simulink model "VCU_SW_1"  (R2023b)
settings: Solver=FixedStepDiscrete  StartTime=0.0  StopTime=inf  FixedStep=1e-2  RelTol=1e-3
PreLoadFcn:
  | RTWConfigurationCB('preloadfcn', bdroot);
InitFcn:
  | loadvar_ttc500
undefined symbols (not defined in the file): BrkPedalTypes, CabMovModeTypes, cFuseTempSensAcc_X, cFuseTempSensAcc_Y, cFuseTempSensVal_X, cFuseTempSensVal_Y, cTMSTempSensVal_X, cTMSTempSensVal_Y, cTransferCaseSpeedRatio, diag_state, DoorsPositionTypes, dP_filter_Y, DriverOccClassSystemTypes, ErrorValueTypes, fatal_error_callback, IO_ADC_NO_RANGE, LadderStatusTypes, pAnalogCabRotSensAcc, pAnalogCabRotSensMaxVolt, pAnalogCabRotSensMinVolt, pAnalogCabRotSensRange, pAnalogCabRotSensZeroVolt, pBrkActivePress, pCabTiltSensAcc, pCabTiltSensMaxCur, pCabTiltSensMinCur, pDistanceCorrection, pECANManual_BPNEnable, pECANManual_BPNEnabler_Flag, pFilterSensAccRes, pHDirMaxDiffFrq, pHDirSensHighLvl, pHDirSensLowLvl, pMainGearRatio, pMaxFilterSensRes, pMaxFirstPedalSensValue, pMaxFuseTempSensRes, pMaxPressLoss, pMaxPressSensCurrent, pMaxPressValue, pMaxPressValueHydMotAndPump, pMaxPressValueParkDrain, pMaxSecondPedalSensValue, pMaxTempSensVoltage, pMaxTempValue, pMaxTMSTempSensRes, pMinFilterSensRes, pMinFirstPedalSensValue, pMinFuseTempSensRes, pMinPressLoss, pMinPressSensCurrent, pMinPressValue, pMinSecondPedalSensValue, pMinTempSensVoltage, pMinTempValue, pMinTMSTempSensRes, pMotorRingTeethNum, pPedalSensAccuracyPct, pPedalSensAccuracyVolt, pPressLossTreshhold ... (+20)
libraries: TTlibrary x270, canmsglib x127, simulink x88
(part 12 of 19)

== system VCU_SW_1/InputLayer/InputInterfaces/AnalogInput/AIProc10msec/WasherTiltPumpTrans ==
  Abs : Abs  SaturateOnIntegerOverflow=off
  Constant12 : Constant  Value=pWasherTiltPumpTransSensMaxVolt
  Constant13 : Constant  Value=pWasherTiltPumpTransSensMinVolt
  Constant14 : Constant  Value=pWasherTiltPumpTransSensAcc
  Data Store Read3 : DataStoreRead  DataStoreName=InputInterfaceData  DataStoreElements=InputInterfaceData.AI.washerTiltPumpTransSens  IndexOptions=Index vector (dialog)  Indices=1  OutputSizes=1
  Data Store Write14 : DataStoreWrite  DataStoreName=InputFunctionsData  DataStoreElements=InputFunctionsData.washerTiltPumpTransPct  IndexOptions=Index vector (dialog)  Indices=1  OutputSizes=1
  Data Store Write40 : DataStoreWrite  DataStoreName=UDSStruct  DataStoreElements=UDSStruct.washerTiltPumpTransSens  IndexOptions=Index vector (dialog)  Indices=1  OutputSizes=1
  Data Type Conversion : DataTypeConversion  OutDataTypeStr=uint16  SaturateOnIntegerOverflow=off  RndMeth=Floor
  getWasherTiltPumpTransSensDataFcn : MATLAB Function  TreatAsAtomicUnit=on
  wires:
  Data Type Conversion/1 -> Data Store Write40/1
  Abs/1 -> Data Type Conversion/1
  getWasherTiltPumpTransSensDataFcn/1(washerTiltPercent) -> Abs/1, Data Store Write14/1
  Constant13/1 -> getWasherTiltPumpTransSensDataFcn/3(minVolt)
  Constant14/1 -> getWasherTiltPumpTransSensDataFcn/4(accuracy)
  Constant12/1 -> getWasherTiltPumpTransSensDataFcn/2(maxVolt)
  Data Store Read3/1 -> getWasherTiltPumpTransSensDataFcn/1(washerTiltPumpTransSens)

== system VCU_SW_1/InputLayer/InputInterfaces/DigitalInput/Function-Call Subsystem/cabRotIndSensProc ==
  function : TriggerPort  TriggerType=function-call  VariantControl=Variant
  Constant1 : Constant  Value=pResetIndCabSensErr
  cabRotIndSensProc fcn : MATLAB Function  TreatAsAtomicUnit=on
  getIndRotSensData : Subsystem  TreatAsAtomicUnit=on
  setIndRotSensData : Subsystem  TreatAsAtomicUnit=on
  setIndSensErr : Subsystem  TreatAsAtomicUnit=on
  wires:
  Constant1/1 -> cabRotIndSensProc fcn/1(pResetIndCabSensErr)

== system VCU_SW_1/InputLayer/InputInterfaces/DigitalInput/Function-Call Subsystem2/cabRotIndSensProc ==
  function : TriggerPort  TriggerType=function-call  VariantControl=Variant
  Constant1 : Constant  Value=pResetIndCabSensErr
  cabRotIndSensProc fcn : MATLAB Function  TreatAsAtomicUnit=on
  getIndRotSensData : Subsystem  TreatAsAtomicUnit=on
  setIndRotSensData : Subsystem  TreatAsAtomicUnit=on
  setIndSensErr : Subsystem  TreatAsAtomicUnit=on
  wires:
  Constant1/1 -> cabRotIndSensProc fcn/1(pResetIndCabSensErr)

== system VCU_SW_1/InputLayer/InputInterfaces/PWDInput/PWDProc100msec/calcSpdSens ==
  calcSpdSensValue : TriggerPort  TriggerType=function-call  IsSimulinkFunction=on  FunctionName=calcSpdSensValue  FunctionVisibility=scoped  VariantControl=(inherit)
  MATLAB Function : MATLAB Function  TreatAsAtomicUnit=on
  teethNum : ArgIn  OutDataTypeStr=uint16  ArgumentName=teethNum
  sensFreq : ArgIn  Port=2  OutDataTypeStr=uint16  ArgumentName=sensFreq
  SpdValue : ArgOut  DisableCoverage=on  OutDataTypeStr=uint16  ArgumentName=SpdValue
  wires:
  sensFreq/1 -> MATLAB Function/1(sensFreq)
  teethNum/1 -> MATLAB Function/2(teethNum)
  MATLAB Function/1(Spd) -> SpdValue/1

== system VCU_SW_1/InputLayer/InputInterfaces/PWDInput/PWDProc100msec/validatePedalSensValue ==
  validateSpdSensValue : TriggerPort  TriggerType=function-call  IsSimulinkFunction=on  FunctionName=validateSpdSensValue  FunctionVisibility=scoped  VariantControl=(inherit)
  Ground : Ground
  MATLAB Function : MATLAB Function  TreatAsAtomicUnit=on
  fstValue : ArgIn  DisableCoverage=on  OutDataTypeStr=uint16  ArgumentName=fstValue
  secValue : ArgIn  Port=2  OutDataTypeStr=uint16  ArgumentName=secValue
  SpdVal : ArgOut  OutDataTypeStr=uint16  ArgumentName=SpdVal
  errorSts : ArgOut  Port=2  OutDataTypeStr=uint8  ArgumentName=errorSts
  wires:
  fstValue/1 -> MATLAB Function/1(firstSensValue)
  secValue/1 -> MATLAB Function/2(secondSensValue)
  Ground/1 -> errorSts/1
  MATLAB Function/1(SpdValue) -> SpdVal/1

== system VCU_SW_1/InputLayer/InputInterfaces/PWMCurrentInput/PWMCur10msecProc/Simulink Function ==
  ValveCurFBproc : TriggerPort  TriggerType=function-call  IsSimulinkFunction=on  FunctionName=ValveCurFBproc  FunctionVisibility=scoped  VariantControl=(inherit)
  MATLAB Function : MATLAB Function  TreatAsAtomicUnit=on
  pValveActiveCur : ArgIn  DisableCoverage=on  OutDataTypeStr=uint16  ArgumentName=pValveActiveCur
  curFB : ArgIn  Port=2  OutDataTypeStr=uint16  ArgumentName=curFB
  stt : ArgOut  DisableCoverage=on  OutDataTypeStr=Enum: StateModeTypes  ArgumentName=stt
  wires:
  MATLAB Function/1(stt) -> stt/1
  curFB/1 -> MATLAB Function/2(curFB)
  pValveActiveCur/1 -> MATLAB Function/1(pValveActiveCur)

== system VCU_SW_1/InputLayer/InputNetwork/InputCCAN/CCAN100msecProc1/CabMov buttons processing ==
  note: Main Fcns
  MATLAB Function : MATLAB Function  TreatAsAtomicUnit=on
  callRotFcn : Subsystem  TreatAsAtomicUnit=on
  callTiltFcn : Subsystem  TreatAsAtomicUnit=on

== system VCU_SW_1/InputLayer/InputNetwork/InputCCAN/CCAN100msecProc1/InputTransSelect ==
  Constant : Constant  Commented=on  Value=3  OutDataTypeStr=uint8
  Constant1 : Constant  Commented=on  Value=0  OutDataTypeStr=uint8
  Constant2 : Constant  Commented=on  Value=0  OutDataTypeStr=uint8
  Constant3 : Constant  Commented=on  OutDataTypeStr=uint8
  Data Store Read : DataStoreRead  DataStoreName=InputNetworkData  DataStoreElements=InputNetworkData.CCAN.TC1.Trans_Requested_Gear  IndexOptions=Index vector (dialog)  Indices=1  OutputSizes=1
  Data Store Read1 : DataStoreRead  DataStoreName=InputInterfaceData  DataStoreElements=InputInterfaceData.DI.selector_signal_1#InputInterfaceData.DI.selector_signal_2#InputInterfaceData.DI.selector_signal_3  IndexOptions=Index vector (dialog)  Indices=1  OutputSizes=1
  Data Store Write1 : DataStoreWrite  DataStoreName=InputFunctionsData  DataStoreElements=InputFunctionsData.LeverPosition  IndexOptions=Index vector (dialog)  Indices=1  OutputSizes=1
  Data Type Conversion : DataTypeConversion  Commented=on  OutDataTypeStr=Enum: StateModeTypes  SaturateOnIntegerOverflow=off  RndMeth=Floor
  Data Type Conversion1 : DataTypeConversion  Commented=on  OutDataTypeStr=Enum: StateModeTypes  SaturateOnIntegerOverflow=off  RndMeth=Floor
  Data Type Conversion2 : DataTypeConversion  Commented=on  OutDataTypeStr=Enum: StateModeTypes  SaturateOnIntegerOverflow=off  RndMeth=Floor
  Data Type Conversion3 : DataTypeConversion  Commented=on  OutDataTypeStr=Enum: LeverPosTypes  SaturateOnIntegerOverflow=off  RndMeth=Floor
  Function Caller1 : FunctionCaller  FunctionPrototype=LeverPos = calcLeverPos(TransReqGear,SelSig1,SelSig2,SelSig3)  InputArgumentSpecifications=<Enter example>  OutputArgumentSpecifications=<Enter example>
  calcLeverPos : Subsystem  TreatAsAtomicUnit=on
  wires:
  Data Store Read1/3 -> Function Caller1/4
  Data Store Read1/2 -> Function Caller1/3
  Data Store Read1/1 -> Function Caller1/2
  Data Store Read/1 -> Function Caller1/1
  Constant3/1 -> Data Type Conversion2/1
  Constant2/1 -> Data Type Conversion1/1
  Constant1/1 -> Data Type Conversion/1
  Constant/1 -> Data Type Conversion3/1
  Function Caller1/1 -> Data Store Write1/1

== system VCU_SW_1/InputLayer/InputNetwork/InputCCAN/CCAN100msecProc1/JoystickRot ==
  Data Store Read1 : DataStoreRead  DataStoreName=InputNetworkData  DataStoreElements=InputNetworkData.CCAN.BJM2.J2_Y_NeutralPosSts#InputNetworkData.CCAN.BJM2.J2_Y_BackNegPosSts#InputNetworkData.CCAN.BJM2.J2_Y_ForwPosSts#InputNetworkData.CCAN.BJM2.J2_Y_Pos  IndexOptions=Index vector (dialog)  Indices=1  OutputSizes=1
  Data Store Write1 : DataStoreWrite  DataStoreName=InputFunctionsData  DataStoreElements=InputFunctionsData.rotJoyPos  IndexOptions=Index vector (dialog)  Indices=1  OutputSizes=1
  Data Store Write2 : DataStoreWrite  DataStoreName=InputFunctionsData  DataStoreElements=InputFunctionsData.rotJoyDir  IndexOptions=Index vector (dialog)  Indices=1  OutputSizes=1
  MATLAB Function : MATLAB Function  TreatAsAtomicUnit=on
  wires:
  MATLAB Function/1(pos) -> Data Store Write1/1
  MATLAB Function/2(dir) -> Data Store Write2/1
  Data Store Read1/1 -> MATLAB Function/1(neutralPos)
  Data Store Read1/2 -> MATLAB Function/2(fwdPos)
  Data Store Read1/4 -> MATLAB Function/4(absPos)
  Data Store Read1/3 -> MATLAB Function/3(bckwsPos)

== system VCU_SW_1/InputLayer/InputNetwork/InputCCAN/GetCCAN1000msec/DD ==
  CAN_Unpack_PLC_StateM : canmsglib/CAN Unpack  MsgList=(none)  MsgName=DD  MsgIDType=Extended (29-bit identifier)  MsgIdentifier=419364094  MsgLength=8  SignalInfo={ 'FuelLevelTank1', '8', '8', 'LE', 'unsigned', 'Standard', '0', '0.4', '0', '0', '100'; 'FuelLevelTank2', '48', '8', 'LE', 'unsigned', 'Standard', '0', '0.4', '0', '0', '100'; 'WasherFluidLevel', '0', '8', 'LE', 'unsigned', 'Standard', '0', '0.4', '0', '0', '100' }  IDPort=off  TimestampPort=off  ErrorPort=off  RemotePort=off  LengthPort=off  StatusPort=off  ApplyMinMax=off
  DataStoreWrite_PLC_StateM : DataStoreWrite  DataStoreName=InputNetworkData  DataStoreElements=InputNetworkData.CCAN.DD.FuelLevelTank1#InputNetworkData.CCAN.DD.FuelLevelTank2#InputNetworkData.CCAN.DD.WasherFluidLevel  IndexOptions=Index vector (dialog)  Indices=1  OutputSizes=1
  Terminator : Terminator
  read_message_PLC_StateM : TTlibrary/CAN/read_message_name  channel=IO_CAN_CHANNEL_1  id_format=IO_CAN_EXT_FRAME  get_msg_info=off  message_names=there is no CAN Unpack blocks  message_info=|  id=419364094  ac_mask=536870911  retranslation=off  io_error=on  sample_time=-1
      | Message Name: DD
      |  Message ID Type: Extended (29-bit identifier)
      |  Message ID: 419364094
      settings: SourceProductName=TT control 500 series
  wires:
  read_message_PLC_StateM/2 -> Terminator/1  "handler_err_419364094"
  read_message_PLC_StateM/1 -> CAN_Unpack_PLC_StateM/1  "msg_419364094"
  CAN_Unpack_PLC_StateM/1 -> DataStoreWrite_PLC_StateM/1
  CAN_Unpack_PLC_StateM/2 -> DataStoreWrite_PLC_StateM/2
  CAN_Unpack_PLC_StateM/3 -> DataStoreWrite_PLC_StateM/3

== system VCU_SW_1/InputLayer/InputNetwork/InputCCAN/GetCCAN1000msec/Fuel Heater Data  ==
  CAN_Unpack_PLC_StateM : canmsglib/CAN Unpack  MsgList=(none)  MsgName=FuelHeaterData  MsgIDType=Extended (29-bit identifier)  MsgIdentifier=419377406  MsgLength=8  SignalInfo={ 'FuelHeaterValue', '0', '8', 'LE', 'unsigned', 'Standard', '0', '0.4', '0', '0', '100' }  IDPort=off  TimestampPort=off  ErrorPort=off  RemotePort=off  LengthPort=off  StatusPort=off  ApplyMinMax=off
  DataStoreWrite_PLC_StateM : DataStoreWrite  DataStoreName=InputNetworkData  DataStoreElements=InputNetworkData.CCAN.FuelHeaterData.FuelHeaterValue  IndexOptions=Index vector (dialog)  Indices=1  OutputSizes=1
  Terminator : Terminator
  read_message_PLC_StateM : TTlibrary/CAN/read_message_name  channel=IO_CAN_CHANNEL_1  id_format=IO_CAN_EXT_FRAME  get_msg_info=off  message_names=there is no CAN Unpack blocks  message_info=|  id=419377406  ac_mask=536870911  retranslation=off  io_error=on  sample_time=-1
      | Message Name: FuelHeaterData
      |  Message ID Type: Extended (29-bit identifier)
      |  Message ID: 419377406
      settings: SourceProductName=TT control 500 series
  wires:
  read_message_PLC_StateM/2 -> Terminator/1  "handler_err_419377406"
  read_message_PLC_StateM/1 -> CAN_Unpack_PLC_StateM/1  "msg_419377406"
  CAN_Unpack_PLC_StateM/1 -> DataStoreWrite_PLC_StateM/1

== system VCU_SW_1/InputLayer/InputNetwork/InputCCAN/GetCCAN1000msec/LCMD ==
  CAN_Unpack_PLC_StateM : canmsglib/CAN Unpack  MsgList=(none)  MsgName=LCMD  MsgIDType=Extended (29-bit identifier)  MsgIdentifier=217989381  MsgLength=8  SignalInfo={ 'CenterStopLightCmd', '18', '2', 'LE', 'unsigned', 'Standard', '0', '1', '0', '0', '3'; 'HighBeamHeadLightCmd', '6', '2', 'LE', 'unsigned', 'Standard', '0', '1', '0', '0', '3'; 'ImplOEMOpt1LightCmd', '50', '2', 'LE', 'unsigned', 'Standard', '0', '1', '0', '0', '3'; 'ImplOEMOpt2LightCmd', '48', '2', 'LE', 'unsigned', 'Standard', '0', '1', '0', '0', '3'; 'ImplRightFacingWrkLightCmd', '52', '2', 'LE', 'unsigned', 'Standard', '0', '1', '0', '0', '3'; 'ImplementMarkerLightCmd', '28', '2', 'LE', 'unsigned', 'Standard', '0', '1', '0', '0', '3'; 'LeftStopLightCmd', '22', '2', 'LE', 'unsigned', 'Standard', '0', '1', '0', '0', '3'; 'LeftTurnSignalLightsCmd', '14', '2', 'LE', 'unsigned', 'Standard', '0', '1', '0', '0', '3'; 'LowBeamHeadLightCmd', '4', '2', 'LE', 'unsigned', 'Standard', '0', '1', '0', '0', '3'; 'RightStopLightCmd', '20', '2', 'LE', 'unsigned', 'Standard', '0', '1', '0', '0', '3'; 'RightTurnSignalLightsCmd', '12', '2', 'LE', 'unsigned', 'Standard', '0', '1', '0', '0', '3'; 'RotatingBeaconLightCmd', '10', '2', 'LE', 'unsigned', 'Standard', '0', '1', '0', '0', '3'; 'RunLightCmd', '0', '2', 'LE', 'unsigned', 'Standard', '0', '1', '0', '0', '3'; 'TractorFrontFogLightsCmd', '8', '2', 'LE', 'unsigned', 'Standard', '0', '1', '0', '0', '3'; 'TrctrFrntHighMntdWrkLightsCmd', '46', '2', 'LE', 'unsigned', 'Standard', '0', '1', '0', '0', '3'; 'TrctrRearHighMntdWrkLightsCmd', '38', '2', 'LE', 'unsigned', 'Standard', '0', '1', '0', '0', '3' }  IDPort=off  TimestampPort=off  ErrorPort=off  RemotePort=off  LengthPort=off  StatusPort=off  ApplyMinMax=off
  DataStoreWrite_PLC_StateM : DataStoreWrite  DataStoreName=InputNetworkData  DataStoreElements=InputNetworkData.CCAN.LCMD_in.CenterStopLightCmd#InputNetworkData.CCAN.LCMD_in.HighBeamHeadLightCmd#InputNetworkData.CCAN.LCMD_in.ImplOEMOpt1LightCmd#InputNetworkData.CCAN.LCMD_in.ImplOEMOpt2LightCmd#InputNetworkData.CCAN.LCMD_in.ImplRightFacingWrkLightCmd#InputNetworkData.CCAN.LCMD_in.ImplementMarkerLightCmd#InputNetworkData.CCAN.LCMD_in.LeftStopLightCmd#InputNetworkData.CCAN.LCMD_in.LeftTurnSignalLightsCmd#InputNetworkData.CCAN.LCMD_in.LowBeamHeadLightCmd#InputNetworkData.CCAN.LCMD_in.RightStopLightCmd#InputNetworkData.CCAN.LCMD_in.RightTurnSignalLightsCmd#InputNetworkData.CCAN.LCMD_in.RotatingBeaconLightCmd#InputNetworkData.CCAN.LCMD_in.RunLightCmd#InputNetworkData.CCAN.LCMD_in.TractorFrontFogLightsCmd#InputNetworkData.CCAN.LCMD_in.TrctrFrntHighMntdWrkLightsCmd#InputNetworkData.CCAN.LCMD_in.TrctrRearHighMntdWrkLightsCmd  IndexOptions=Index vector (dialog)  Indices=1  OutputSizes=1
  Function Caller{1..16} (16 alike) : FunctionCaller  FunctionPrototype=rawValue = convUintPinToenumStt(uintValue)  InputArgumentSpecifications=<Enter example>  OutputArgumentSpecifications=<Enter example>
  Terminator : Terminator
  read_message_PLC_StateM : TTlibrary/CAN/read_message_name  channel=IO_CAN_CHANNEL_1  id_format=IO_CAN_EXT_FRAME  get_msg_info=off  message_names=there is no CAN Unpack blocks  message_info=|  id=217989381  ac_mask=536870911  retranslation=off  io_error=on  sample_time=-1
      | Message Name: LCMD
      |  Message ID Type: Extended (29-bit identifier)
      |  Message ID: 217989381
      settings: SourceProductName=TT control 500 series
  wires:
  Function Caller16/1 -> DataStoreWrite_PLC_StateM/16
  Function Caller15/1 -> DataStoreWrite_PLC_StateM/15
  Function Caller14/1 -> DataStoreWrite_PLC_StateM/14
  Function Caller13/1 -> DataStoreWrite_PLC_StateM/13
  Function Caller12/1 -> DataStoreWrite_PLC_StateM/12
  Function Caller11/1 -> DataStoreWrite_PLC_StateM/11
  Function Caller10/1 -> DataStoreWrite_PLC_StateM/10
  Function Caller9/1 -> DataStoreWrite_PLC_StateM/9
  Function Caller8/1 -> DataStoreWrite_PLC_StateM/8
  Function Caller7/1 -> DataStoreWrite_PLC_StateM/7
  Function Caller6/1 -> DataStoreWrite_PLC_StateM/6
  Function Caller5/1 -> DataStoreWrite_PLC_StateM/5
  Function Caller4/1 -> DataStoreWrite_PLC_StateM/4
  Function Caller3/1 -> DataStoreWrite_PLC_StateM/3
  Function Caller2/1 -> DataStoreWrite_PLC_StateM/2
  Function Caller1/1 -> DataStoreWrite_PLC_StateM/1
  CAN_Unpack_PLC_StateM/16 -> Function Caller16/1
  CAN_Unpack_PLC_StateM/15 -> Function Caller15/1
  CAN_Unpack_PLC_StateM/14 -> Function Caller14/1
  CAN_Unpack_PLC_StateM/13 -> Function Caller13/1
  CAN_Unpack_PLC_StateM/12 -> Function Caller12/1
  CAN_Unpack_PLC_StateM/11 -> Function Caller11/1
  CAN_Unpack_PLC_StateM/10 -> Function Caller10/1
  CAN_Unpack_PLC_StateM/9 -> Function Caller9/1
  CAN_Unpack_PLC_StateM/8 -> Function Caller8/1
  CAN_Unpack_PLC_StateM/7 -> Function Caller7/1
  CAN_Unpack_PLC_StateM/6 -> Function Caller6/1
  CAN_Unpack_PLC_StateM/5 -> Function Caller5/1
  CAN_Unpack_PLC_StateM/4 -> Function Caller4/1
  CAN_Unpack_PLC_StateM/3 -> Function Caller3/1
  CAN_Unpack_PLC_StateM/2 -> Function Caller2/1
  read_message_PLC_StateM/2 -> Terminator/1  "handler_err_217989381"
  read_message_PLC_StateM/1 -> CAN_Unpack_PLC_StateM/1  "msg_217989381"
  CAN_Unpack_PLC_StateM/1 -> Function Caller1/1

== system VCU_SW_1/InputLayer/InputNetwork/InputCCAN/GetCCAN1000msec/LD ==
  CAN_Unpack_PLC_StateM : canmsglib/CAN Unpack  MsgList=(none)  MsgName=LD  MsgIDType=Extended (29-bit identifier)  MsgIdentifier=217989374  MsgLength=8  SignalInfo={ 'CenterStopLight', '18', '2', 'LE', 'unsigned', 'Standard', '0', '1', '0', '0', '3'; 'HighBeamHeadLightData', '6', '2', 'LE', 'unsigned', 'Standard', '0', '1', '0', '0', '3'; 'ImplOEMOpt1Light', '50', '2', 'LE', 'unsigned', 'Standard', '0', '1', '0', '0', '3'; 'ImplOEMOpt2Light', '48', '2', 'LE', 'unsigned', 'Standard', '0', '1', '0', '0', '3'; 'ImplRightFacingWrkLight', '52', '2', 'LE', 'unsigned', 'Standard', '0', '1', '0', '0', '3'; 'ImplementMarkerLight', '28', '2', 'LE', 'unsigned', 'Standard', '0', '1', '0', '0', '3'; 'LeftStopLight', '22', '2', 'LE', 'unsigned', 'Standard', '0', '1', '0', '0', '3'; 'LeftTurnSignalLights', '14', '2', 'LE', 'unsigned', 'Standard', '0', '1', '0', '0', '3'; 'LowBeamHeadLightData', '4', '2', 'LE', 'unsigned', 'Standard', '0', '1', '0', '0', '3'; 'RightStopLight', '20', '2', 'LE', 'unsigned', 'Standard', '0', '1', '0', '0', '3'; 'RightTurnSignalLights', '12', '2', 'LE', 'unsigned', 'Standard', '0', '1', '0', '0', '3'; 'RotatingBeaconLight', '10', '2', 'LE', 'unsigned', 'Standard', '0', '1', '0', '0', '3'; 'RunLight', '0', '2', 'LE', 'unsigned', 'Standard', '0', '1', '0', '0', '3'; 'TractorFrontFogLights', '8', '2', 'LE', 'unsigned', 'Standard', '0', '1', '0', '0', '3'; 'TrctrFrntHighMntdWrkLightsData', '46', '2', 'LE', 'unsigned', 'Standard', '0', '1', '0', '0', '3'; 'TrctrRearHighMntdWrkLightsData', '38', '2', 'LE', 'unsigned', 'Standard', '0', '1', '0', '0', '3' }  IDPort=off  TimestampPort=off  ErrorPort=off  RemotePort=off  LengthPort=off  StatusPort=off  ApplyMinMax=off
  DataStoreWrite_PLC_StateM : DataStoreWrite  DataStoreName=InputNetworkData  DataStoreElements=InputNetworkData.CCAN.LD.CenterStopLight#InputNetworkData.CCAN.LD.HighBeamHeadLightData#InputNetworkData.CCAN.LD.ImplOEMOpt1Light#InputNetworkData.CCAN.LD.ImplOEMOpt2Light#InputNetworkData.CCAN.LD.ImplRightFacingWrkLight#InputNetworkData.CCAN.LD.ImplementMarkerLight#InputNetworkData.CCAN.LD.LeftStopLight#InputNetworkData.CCAN.LD.LeftTurnSignalLights#InputNetworkData.CCAN.LD.LowBeamHeadLightData#InputNetworkData.CCAN.LD.RightStopLight#InputNetworkData.CCAN.LD.RightTurnSignalLights#InputNetworkData.CCAN.LD.RotatingBeaconLight#InputNetworkData.CCAN.LD.RunLight#InputNetworkData.CCAN.LD.TractorFrontFogLights#InputNetworkData.CCAN.LD.TrctrFrntHighMntdWrkLightsData#InputNetworkData.CCAN.LD.TrctrRearHighMntdWrkLightsData  IndexOptions=Index vector (dialog)  Indices=1  OutputSizes=1
  Terminator : Terminator
  read_message_PLC_StateM : TTlibrary/CAN/read_message_name  channel=IO_CAN_CHANNEL_1  id_format=IO_CAN_EXT_FRAME  get_msg_info=off  message_names=there is no CAN Unpack blocks  message_info=|  id=217989374  ac_mask=536870911  retranslation=off  io_error=on  sample_time=-1
      | Message Name: LD
      |  Message ID Type: Extended (29-bit identifier)
      |  Message ID: 217989374
      settings: SourceProductName=TT control 500 series
  wires:
  CAN_Unpack_PLC_StateM/6 -> DataStoreWrite_PLC_StateM/6
  CAN_Unpack_PLC_StateM/5 -> DataStoreWrite_PLC_StateM/5
  CAN_Unpack_PLC_StateM/4 -> DataStoreWrite_PLC_StateM/4
  CAN_Unpack_PLC_StateM/3 -> DataStoreWrite_PLC_StateM/3
  CAN_Unpack_PLC_StateM/2 -> DataStoreWrite_PLC_StateM/2
  CAN_Unpack_PLC_StateM/1 -> DataStoreWrite_PLC_StateM/1
  read_message_PLC_StateM/2 -> Terminator/1  "handler_err_217989374"
  read_message_PLC_StateM/1 -> CAN_Unpack_PLC_StateM/1  "msg_217989374"
  CAN_Unpack_PLC_StateM/7 -> DataStoreWrite_PLC_StateM/7
  CAN_Unpack_PLC_StateM/8 -> DataStoreWrite_PLC_StateM/8
  CAN_Unpack_PLC_StateM/9 -> DataStoreWrite_PLC_StateM/9
  CAN_Unpack_PLC_StateM/10 -> DataStoreWrite_PLC_StateM/10
  CAN_Unpack_PLC_StateM/11 -> DataStoreWrite_PLC_StateM/11
  CAN_Unpack_PLC_StateM/12 -> DataStoreWrite_PLC_StateM/12
  CAN_Unpack_PLC_StateM/13 -> DataStoreWrite_PLC_StateM/13
  CAN_Unpack_PLC_StateM/14 -> DataStoreWrite_PLC_StateM/14
  CAN_Unpack_PLC_StateM/15 -> DataStoreWrite_PLC_StateM/15
  CAN_Unpack_PLC_StateM/16 -> DataStoreWrite_PLC_StateM/16

== system VCU_SW_1/InputLayer/InputNetwork/InputCCAN/GetCCAN1000msec/OCSI ==
  CAN_Unpack_PLC_StateM : canmsglib/CAN Unpack  MsgList=(none)  MsgName=OCSI  MsgIDType=Extended (29-bit identifier)  MsgIdentifier=419239678  MsgLength=8  SignalInfo={ 'DrvrOccClassSysSts', '0', '3', 'LE', 'unsigned', 'Standard', '0', '1', '0', '0', '7' }  IDPort=off  TimestampPort=off  ErrorPort=off  RemotePort=off  LengthPort=off  StatusPort=off  ApplyMinMax=off
  DataStoreWrite_PLC_StateM : DataStoreWrite  DataStoreName=InputNetworkData  DataStoreElements=InputNetworkData.CCAN.OCSI.DrvrOccClassSysSts  IndexOptions=Index vector (dialog)  Indices=1  OutputSizes=1
  Enumerated Constant4 : simulink/Sources/Enumerated Constant  OutDataTypeStr=Enum: DriverOccClassSystemTypes  Value=DriverOccClassSystemTypes.DRIVER_CLASS_DRIVER_PRESENT  SampleTime=inf
  MATLAB Function : MATLAB Function  TreatAsAtomicUnit=on
  Terminator : Terminator
  read_message_PLC_StateM : TTlibrary/CAN/read_message_name  channel=IO_CAN_CHANNEL_1  id_format=IO_CAN_EXT_FRAME  get_msg_info=off  message_names=there is no CAN Unpack blocks  message_info=|  id=419239678  ac_mask=536870911  retranslation=off  io_error=on  sample_time=-1
      | Message Name: OCSI
      |  Message ID Type: Extended (29-bit identifier)
      |  Message ID: 419239678
      settings: SourceProductName=TT control 500 series
  wires:
  Enumerated Constant4/1 -> DataStoreWrite_PLC_StateM/1
  read_message_PLC_StateM/2 -> Terminator/1  "handler_err_419239678"
  read_message_PLC_StateM/1 -> CAN_Unpack_PLC_StateM/1  "msg_419239678"
  CAN_Unpack_PLC_StateM/1 -> MATLAB Function/1(Value)

== system VCU_SW_1/InputLayer/InputNetwork/InputCCAN/GetCCAN1000msec/VF ==
  CAN_Unpack_PLC_StateM : canmsglib/CAN Unpack  MsgList=(none)  MsgName=VF  MsgIDType=Extended (29-bit identifier)  MsgIdentifier=419326206  MsgLength=8  SignalInfo={ 'HydrOilFilterRestrSwtch', '8', '2', 'LE', 'unsigned', 'Standard', '0', '1', '0', '0', '3'; 'HydraulicOilLevel', '16', '8', 'LE', 'unsigned', 'Standard', '0', '0.4', '0', '0', '100'; 'HydraulicTemperature', '0', '8', 'LE', 'unsigned', 'Standard', '0', '1', '-40', '-40', '210' }  IDPort=off  TimestampPort=off  ErrorPort=off  RemotePort=off  LengthPort=off  StatusPort=off  ApplyMinMax=off
  DataStoreWrite_PLC_StateM : DataStoreWrite  DataStoreName=InputNetworkData  DataStoreElements=InputNetworkData.CCAN.VF.HydrOilFilterRestrSwtch#InputNetworkData.CCAN.VF.HydraulicOilLevel#InputNetworkData.CCAN.VF.HydraulicTemperature  IndexOptions=Index vector (dialog)  Indices=1  OutputSizes=1
  Function Caller1 : FunctionCaller  FunctionPrototype=rawValue = convUintPinToenumStt(uintValue)  InputArgumentSpecifications=<Enter example>  OutputArgumentSpecifications=<Enter example>
  Terminator : Terminator
  read_message_PLC_StateM : TTlibrary/CAN/read_message_name  channel=IO_CAN_CHANNEL_1  id_format=IO_CAN_EXT_FRAME  get_msg_info=off  message_names=there is no CAN Unpack blocks  message_info=|  id=419326206  ac_mask=536870911  retranslation=off  io_error=on  sample_time=-1
      | Message Name: VF
      |  Message ID Type: Extended (29-bit identifier)
      |  Message ID: 419326206
      settings: SourceProductName=TT control 500 series
  wires:
  Function Caller1/1 -> DataStoreWrite_PLC_StateM/1
  CAN_Unpack_PLC_StateM/3 -> DataStoreWrite_PLC_StateM/3
  CAN_Unpack_PLC_StateM/2 -> DataStoreWrite_PLC_StateM/2
  read_message_PLC_StateM/2 -> Terminator/1  "handler_err_419326206"
  read_message_PLC_StateM/1 -> CAN_Unpack_PLC_StateM/1  "msg_419326206"
  CAN_Unpack_PLC_StateM/1 -> Function Caller1/1

== system VCU_SW_1/InputLayer/InputNetwork/InputCCAN/GetCCAN100msec/AUX_VLV_EST_CABIN ==
  CAN_Unpack_AUX_VLV_EST_CABIN : canmsglib/CAN Unpack  MsgList=(none)  MsgName=AUX_VLV_EST_CABIN  MsgIDType=Extended (29-bit identifier)  MsgIdentifier=217977217  MsgLength=3  SignalInfo={ 'ExtendPortFlowCabine', '0', '8', 'LE', 'unsigned', 'Standard', '0', '1', '125', '125', '225'; 'FailSafeModeFlowCabine', '22', '2', 'LE', 'unsigned', 'Standard', '0', '1', '0', '0', '3'; 'RetractPortFlowCabine', '8', '8', 'LE', 'unsigned', 'Standard', '0', '1', '125', '125', '225'; 'ValveStateFlowCabine', '16', '4', 'LE', 'unsigned', 'Standard', '0', '1', '0', '0', '15' }  IDPort=off  TimestampPort=off  ErrorPort=off  RemotePort=off  LengthPort=off  StatusPort=off  ApplyMinMax=off
  DataStoreWrite_PLC_StateM : DataStoreWrite  DataStoreName=InputNetworkData  DataStoreElements=InputNetworkData.CCAN.AUX_VLV_EST_CABIN.ExtendPortFlowCabine#InputNetworkData.CCAN.AUX_VLV_EST_CABIN.FailSafeModeFlowCabine#InputNetworkData.CCAN.AUX_VLV_EST_CABIN.RetractPortFlowCabine#InputNetworkData.CCAN.AUX_VLV_EST_CABIN.ValveStateFlowCabine  IndexOptions=Index vector (dialog)  Indices=1  OutputSizes=1
  Terminator : Terminator
  read_message_AUX_VLV_EST_CABIN : TTlibrary/CAN/read_message_name  channel=IO_CAN_CHANNEL_1  id_format=IO_CAN_EXT_FRAME  get_msg_info=off  message_names=there is no CAN Unpack blocks  message_info=|  id=217977217  ac_mask=536870911  retranslation=off  io_error=on  sample_time=-1
      | Message Name: AUX_VLV_EST_CABIN
      |  Message ID Type: Extended (29-bit identifier)
      |  Message ID: 217977217
      settings: SourceProductName=TT control 500 series
  wires:
  read_message_AUX_VLV_EST_CABIN/2 -> Terminator/1  "handler_err_217977217"
  read_message_AUX_VLV_EST_CABIN/1 -> CAN_Unpack_AUX_VLV_EST_CABIN/1  "msg_217977217"
  CAN_Unpack_AUX_VLV_EST_CABIN/1 -> DataStoreWrite_PLC_StateM/1
  CAN_Unpack_AUX_VLV_EST_CABIN/2 -> DataStoreWrite_PLC_StateM/2
  CAN_Unpack_AUX_VLV_EST_CABIN/3 -> DataStoreWrite_PLC_StateM/3
  CAN_Unpack_AUX_VLV_EST_CABIN/4 -> DataStoreWrite_PLC_StateM/4

== system VCU_SW_1/InputLayer/InputNetwork/InputCCAN/GetCCAN100msec/BJM1 ==
  CAN_Unpack_Cab_BJM1 : canmsglib/CAN Unpack  MsgList=(none)  MsgName=BJM1  MsgIDType=Extended (29-bit identifier)  MsgIdentifier=217961989  MsgLength=8  SignalInfo={ 'J1_Bttn_1_PressSts', '46', '2', 'LE', 'unsigned', 'Standard', '0', '1', '0', '0', '3'; 'J1_Bttn_2_PressSts', '44', '2', 'LE', 'unsigned', 'Standard', '0', '1', '0', '0', '3'; 'J1_Bttn_3_PressSts', '42', '2', 'LE', 'unsigned', 'Standard', '0', '1', '0', '0', '3'; 'J1_Bttn_4_PressSts', '40', '2', 'LE', 'unsigned', 'Standard', '0', '1', '0', '0', '3'; 'J1_Bttn_5_PressSts', '54', '2', 'LE', 'unsigned', 'Standard', '0', '1', '0', '0', '3'; 'J1_Bttn_6_PressSts', '52', '2', 'LE', 'unsigned', 'Standard', '0', '1', '0', '0', '3'; 'J1_Bttn_7_PressSts', '50', '2', 'LE', 'unsigned', 'Standard', '0', '1', '0', '0', '3' }  IDPort=off  TimestampPort=off  ErrorPort=off  RemotePort=off  LengthPort=off  StatusPort=off  ApplyMinMax=off
  DataStoreWrite_Str_BJM2 : DataStoreWrite  DataStoreName=InputNetworkData  DataStoreElements=InputNetworkData.CCAN.BJM1.But1CabRollRight#InputNetworkData.CCAN.BJM1.But2CabRollLeft#InputNetworkData.CCAN.BJM1.But3CabPitchFwd#InputNetworkData.CCAN.BJM1.But4CabPitchBckwd#InputNetworkData.CCAN.BJM1.But5CabTiltReturn#InputNetworkData.CCAN.BJM1.But6CabStab#InputNetworkData.CCAN.BJM1.But7CabRotReturn  IndexOptions=Index vector (dialog)  Indices=1  OutputSizes=1
  Function Caller{1..6,9} (7 alike) : FunctionCaller  FunctionPrototype=rawValue = convUintPinToenumStt(uintValue)  InputArgumentSpecifications=<Enter example>  OutputArgumentSpecifications=<Enter example>
  Terminator2 : Terminator
  read_message_Cab_BJM1 : TTlibrary/CAN/read_message_name  channel=IO_CAN_CHANNEL_3  id_format=IO_CAN_EXT_FRAME  get_msg_info=off  message_names=there is no CAN Unpack blocks  message_info=|  id=217961989  ac_mask=536870911  retranslation=off  io_error=on  sample_time=-1
      | Message Name: BJM1
      |  Message ID Type: Extended (29-bit identifier)
      |  Message ID: 419288581
      settings: SourceProductName=TT control 500 series
  wires:
  CAN_Unpack_Cab_BJM1/1 -> Function Caller9/1
  read_message_Cab_BJM1/2 -> Terminator2/1  "handler_err_217961989"
  CAN_Unpack_Cab_BJM1/5 -> Function Caller2/1
  Function Caller9/1 -> DataStoreWrite_Str_BJM2/1
  read_message_Cab_BJM1/1 -> CAN_Unpack_Cab_BJM1/1  "msg_217961989"
  CAN_Unpack_Cab_BJM1/2 -> Function Caller1/1
  CAN_Unpack_Cab_BJM1/3 -> Function Caller3/1
  CAN_Unpack_Cab_BJM1/4 -> Function Caller4/1
  CAN_Unpack_Cab_BJM1/6 -> Function Caller5/1
  CAN_Unpack_Cab_BJM1/7 -> Function Caller6/1
  Function Caller1/1 -> DataStoreWrite_Str_BJM2/2
  Function Caller3/1 -> DataStoreWrite_Str_BJM2/3
  Function Caller4/1 -> DataStoreWrite_Str_BJM2/4
  Function Caller2/1 -> DataStoreWrite_Str_BJM2/5
  Function Caller5/1 -> DataStoreWrite_Str_BJM2/6
  Function Caller6/1 -> DataStoreWrite_Str_BJM2/7

== system VCU_SW_1/InputLayer/InputNetwork/InputCCAN/GetCCAN100msec/BJM2 ==
  note: Выпилить эти переменные из структуры, заменить названия на те, что будут после обработки. Получается, что из структур, в которые сейчас пишутся обработанные данные (InputFunctions) их тоже надо выпилить, с переносом в структуру InputNetwork.CCAN.BJM2
  CAN_Unpack_Cab_BJM2 : canmsglib/CAN Unpack  MsgList=(none)  MsgName=BJM2  MsgIDType=Extended (29-bit identifier)  MsgIdentifier=217962501  MsgLength=8  SignalInfo={ 'J2_X_LeftNegPosSts', '2', '2', 'LE', 'unsigned', 'Standard', '0', '1', '0', '0', '3'; 'J2_X_NeutralPosSts', '0', '2', 'LE', 'unsigned', 'Standard', '0', '1', '0', '0', '3'; 'J2_X_Pos', '6', '10', 'LE', 'unsigned', 'Standard', '0', '0.1', '0', '0', '102'; 'J2_X_RightPosSts', '4', '2', 'LE', 'unsigned', 'Standard', '0', '1', '0', '0', '3'; 'J2_Y_BackNegPosSts', '18', '2', 'LE', 'unsigned', 'Standard', '0', '1', '0', '0', '3'; 'J2_Y_ForwPosSts', '20', '2', 'LE', 'unsigned', 'Standard', '0', '1', '0', '0', '3'; 'J2_Y_NeutralPosSts', '16', '2', 'LE', 'unsigned', 'Standard', '0', '1', '0', '0', '3'; 'J2_Y_Pos', '22', '10', 'LE', 'unsigned', 'Standard', '0', '0.1', '0', '0', '102' }  IDPort=off  TimestampPort=off  ErrorPort=off  RemotePort=off  LengthPort=off  StatusPort=off  ApplyMinMax=off
  DataStoreWrite_PLC_StateM : DataStoreWrite  DataStoreName=InputNetworkData  DataStoreElements=InputNetworkData.CCAN.BJM2.J2_Y_BackNegPosSts#InputNetworkData.CCAN.BJM2.J2_Y_ForwPosSts#InputNetworkData.CCAN.BJM2.J2_Y_NeutralPosSts#InputNetworkData.CCAN.BJM2.J2_Y_Pos  IndexOptions=Index vector (dialog)  Indices=1  OutputSizes=1
  Function Caller1 : FunctionCaller  FunctionPrototype=rawValue = convUintPinToenumStt(uintValue)  InputArgumentSpecifications=<Enter example>  OutputArgumentSpecifications=<Enter example>
  Function Caller2 : FunctionCaller  FunctionPrototype=rawValue = convUintPinToenumStt(uintValue)  InputArgumentSpecifications=<Enter example>  OutputArgumentSpecifications=<Enter example>
  Function Caller7 : FunctionCaller  FunctionPrototype=rawValue = convUintPinToenumStt(uintValue)  InputArgumentSpecifications=<Enter example>  OutputArgumentSpecifications=<Enter example>
  Terminator{,1..4} (5 alike) : Terminator
  read_message_Cab_BJM2 : TTlibrary/CAN/read_message_name  channel=IO_CAN_CHANNEL_1  id_format=IO_CAN_EXT_FRAME  get_msg_info=off  message_names=there is no CAN Unpack blocks  message_info=|  id=217962501  ac_mask=536870911  retranslation=off  io_error=on  sample_time=-1
      | Message Name: BJM2
      |  Message ID Type: Extended (29-bit identifier)
      |  Message ID: 217962501
      settings: SourceProductName=TT control 500 series
  wires:
  read_message_Cab_BJM2/1 -> CAN_Unpack_Cab_BJM2/1  "msg_217962501"
  read_message_Cab_BJM2/2 -> Terminator/1  "handler_err_217962501"
  CAN_Unpack_Cab_BJM2/5 -> Function Caller1/1
  CAN_Unpack_Cab_BJM2/6 -> Function Caller7/1
  CAN_Unpack_Cab_BJM2/7 -> Function Caller2/1
  CAN_Unpack_Cab_BJM2/4 -> Terminator1/1
  CAN_Unpack_Cab_BJM2/3 -> Terminator2/1
  CAN_Unpack_Cab_BJM2/2 -> Terminator3/1
  CAN_Unpack_Cab_BJM2/1 -> Terminator4/1
  CAN_Unpack_Cab_BJM2/8 -> DataStoreWrite_PLC_StateM/4
  Function Caller2/1 -> DataStoreWrite_PLC_StateM/3
  Function Caller7/1 -> DataStoreWrite_PLC_StateM/2
  Function Caller1/1 -> DataStoreWrite_PLC_StateM/1

== system VCU_SW_1/InputLayer/InputNetwork/InputCCAN/GetCCAN100msec/CM1 ==
  note: Команда идет наоборот, какого хера тут было это?
  CAN_Unpack_Cab_CM1 : canmsglib/CAN Unpack  MsgList=(none)  MsgName=CM1  MsgIDType=Extended (29-bit identifier)  MsgIdentifier=417397253  MsgLength=5  SignalInfo={ 'Park_Brake_Command', '32', '2', 'LE', 'unsigned', 'Standard', '0', '1', '0', '0', '3' }  IDPort=off  TimestampPort=off  ErrorPort=off  RemotePort=off  LengthPort=off  StatusPort=off  ApplyMinMax=off
  Constant : Constant  Value=uint8(1)
  DataStoreWrite_PLC_StateM : DataStoreWrite  DataStoreName=InputNetworkData  DataStoreElements=InputNetworkData.CCAN.CM1.Park_Brake_Command  IndexOptions=Index vector (dialog)  Indices=1  OutputSizes=1
  Enumerated Constant : simulink/Sources/Enumerated Constant  OutDataTypeStr=Enum: StateModeTypes  Value=StateModeTypes.STT_DISABLE  SampleTime=inf
  Enumerated Constant1 : simulink/Sources/Enumerated Constant  OutDataTypeStr=Enum: StateModeTypes  Value=StateModeTypes.STT_ENABLE  SampleTime=inf
  Function Caller1 : FunctionCaller  Commented=on  FunctionPrototype=rawValue = convUintPinToenumStt(uintValue)  InputArgumentSpecifications=<Enter example>  OutputArgumentSpecifications=<Enter example>
  Multiport Switch : MultiPortSwitch  DataPortOrder=Zero-based contiguous  Inputs=2  zeroidx=on  SaturateOnIntegerOverflow=off  InputSameDT=off
  Relational Operator : RelationalOperator  Operator===  OutDataTypeStr=boolean  RndMeth=Simplest  InputSameDT=off
  Terminator : Terminator
  read_message_Cab_CM1 : TTlibrary/CAN/read_message_name  channel=IO_CAN_CHANNEL_1  id_format=IO_CAN_EXT_FRAME  get_msg_info=off  message_names=there is no CAN Unpack blocks  message_info=|  id=417397253  ac_mask=536870911  retranslation=off  io_error=on  sample_time=-1
      | Message Name: CM1
      |  Message ID Type: Extended (29-bit identifier)
      |  Message ID: 417397253
      settings: SourceProductName=TT control 500 series
  wires:
  read_message_Cab_CM1/1 -> CAN_Unpack_Cab_CM1/1  "msg_417397253"
  read_message_Cab_CM1/2 -> Terminator/1  "handler_err_417397253"
  CAN_Unpack_Cab_CM1/1 -> Relational Operator/1
  Constant/1 -> Relational Operator/2
  Relational Operator/1 -> Multiport Switch/1
  Enumerated Constant1/1 -> Multiport Switch/2
  Enumerated Constant/1 -> Multiport Switch/3
  Multiport Switch/1 -> DataStoreWrite_PLC_StateM/1

== system VCU_SW_1/InputLayer/InputNetwork/InputCCAN/GetCCAN100msec/CM3 ==
  CAN_Unpack_Cab_CM3 : canmsglib/CAN Unpack  MsgList=(none)  MsgName=CM3  MsgIDType=Extended (29-bit identifier)  MsgIdentifier=419288069  MsgLength=8  SignalInfo={ 'Transfer_Case_Selector_Switch', '0', '3', 'LE', 'unsigned', 'Standard', '0', '1', '0', '0', '7' }  IDPort=off  TimestampPort=off  ErrorPort=off  RemotePort=off  LengthPort=off  StatusPort=off  ApplyMinMax=off
  DataStoreWrite_PLC_StateM : DataStoreWrite  DataStoreName=InputNetworkData  DataStoreElements=InputNetworkData.CCAN.CM3.Transfer_Case_Selector_Switch  IndexOptions=Index vector (dialog)  Indices=1  OutputSizes=1
  MATLAB Function : MATLAB Function  TreatAsAtomicUnit=on
  Terminator : Terminator
  read_message_Cab_CM3 : TTlibrary/CAN/read_message_name  channel=IO_CAN_CHANNEL_1  id_format=IO_CAN_EXT_FRAME  get_msg_info=off  message_names=there is no CAN Unpack blocks  message_info=|  id=419288069  ac_mask=536870911  retranslation=off  io_error=on  sample_time=-1
      | Message Name: CM3
      |  Message ID Type: Extended (29-bit identifier)
      |  Message ID: 419288069
      settings: SourceProductName=TT control 500 series
  wires:
  MATLAB Function/1(TransferCaseEnum) -> DataStoreWrite_PLC_StateM/1
  CAN_Unpack_Cab_CM3/1 -> MATLAB Function/1(value)
  read_message_Cab_CM3/1 -> CAN_Unpack_Cab_CM3/1  "msg_419288069"
  read_message_Cab_CM3/2 -> Terminator/1  "handler_err_419288069"

== system VCU_SW_1/InputLayer/InputNetwork/InputCCAN/GetCCAN100msec/CabinAuxiliaryStatus ==
  CAN_Unpack_CabinAuxiliaryStatus : canmsglib/CAN Unpack  MsgList=(none)  MsgName=CabinAuxiliaryStatus  MsgIDType=Extended (29-bit identifier)  MsgIdentifier=419376638  MsgLength=8  SignalInfo={ 'FrameLockSts', '2', '2', 'LE', 'unsigned', 'Standard', '0', '1', '0', '0', '3'; 'FuelTankStatus', '0', '2', 'LE', 'unsigned', 'Standard', '0', '1', '0', '0', '3'; 'LadderStatus', '4', '2', 'LE', 'unsigned', 'Standard', '0', '1', '0', '0', '3' }  IDPort=off  TimestampPort=off  ErrorPort=off  RemotePort=off  LengthPort=off  StatusPort=off  ApplyMinMax=off
  DataStoreWrite_PLC_StateM : DataStoreWrite  DataStoreName=InputNetworkData  DataStoreElements=InputNetworkData.CCAN.CabinAuxiliaryStatus.FrameLockStatus#InputNetworkData.CCAN.CabinAuxiliaryStatus.FuelTankStatus#InputNetworkData.CCAN.CabinAuxiliaryStatus.LadderStatus  IndexOptions=Index vector (dialog)  Indices=1  OutputSizes=1
  Enumerated Constant1 : simulink/Sources/Enumerated Constant  OutDataTypeStr=Enum: StateModeTypes  Value=StateModeTypes.STT_DISABLE  SampleTime=inf
  Enumerated Constant8 : simulink/Sources/Enumerated Constant  OutDataTypeStr=Enum: LadderStatusTypes  Value=LadderStatusTypes.LADDER_UP  SampleTime=inf
  Function Caller1 : FunctionCaller  FunctionPrototype=rawValue = convUintPinToenumStt(uintValue)  InputArgumentSpecifications=<Enter example>  OutputArgumentSpecifications=<Enter example>
  Function Caller3 : FunctionCaller  FunctionPrototype=rawValue = convUintPinToenumStt(uintValue)  InputArgumentSpecifications=<Enter example>  OutputArgumentSpecifications=<Enter example>
  MATLAB Function : MATLAB Function  TreatAsAtomicUnit=on
  Terminator : Terminator
  read_message_CabinAuxiliaryStatus : TTlibrary/CAN/read_message_name  channel=IO_CAN_CHANNEL_1  id_format=IO_CAN_EXT_FRAME  get_msg_info=off  message_names=there is no CAN Unpack blocks  message_info=|  id=419376638  ac_mask=536870911  retranslation=off  io_error=on  sample_time=-1
      | Message Name: InstrumentClusterStatus
      |  Message ID Type: Extended (29-bit identifier)
      |  Message ID: 419384087
      settings: SourceProductName=TT control 500 series
  wires:
  read_message_CabinAuxiliaryStatus/2 -> Terminator/1  "handler_err_419376638"
  read_message_CabinAuxiliaryStatus/1 -> CAN_Unpack_CabinAuxiliaryStatus/1  "msg_419376638"
  CAN_Unpack_CabinAuxiliaryStatus/1 -> Function Caller3/1
  CAN_Unpack_CabinAuxiliaryStatus/3 -> MATLAB Function/1(Value)
  CAN_Unpack_CabinAuxiliaryStatus/2 -> Function Caller1/1
  Enumerated Constant1/1 -> DataStoreWrite_PLC_StateM/1
  Function Caller1/1 -> DataStoreWrite_PLC_StateM/2
  Enumerated Constant8/1 -> DataStoreWrite_PLC_StateM/3

== system VCU_SW_1/InputLayer/InputNetwork/InputCCAN/GetCCAN100msec/DC1 ==
  CAN_Unpack_Cab_DC1 : canmsglib/CAN Unpack  MsgList=(none)  MsgName=DC1  MsgIDType=Extended (29-bit identifier)  MsgIdentifier=419319550  MsgLength=8  SignalInfo={ 'PositionOfDoors', '0', '4', 'LE', 'unsigned', 'Standard', '0', '1', '0', '0', '15' }  IDPort=off  TimestampPort=off  ErrorPort=off  RemotePort=off  LengthPort=off  StatusPort=off  ApplyMinMax=off
  Data Store Write : DataStoreWrite  DataStoreName=InputFunctionsData  DataStoreElements=InputFunctionsData.doorIsClosed  IndexOptions=Index vector (dialog)  Indices=1  OutputSizes=1
  DataStoreWrite_PLC_StateM : DataStoreWrite  DataStoreName=InputNetworkData  DataStoreElements=InputNetworkData.CCAN.DC1.PositionOfDoors  IndexOptions=Index vector (dialog)  Indices=1  OutputSizes=1
  Enumerated Constant : simulink/Sources/Enumerated Constant  OutDataTypeStr=Enum: DoorsPositionTypes  Value=DoorsPositionTypes.DOORS_POS_ALL_DOORS_CLOSED  SampleTime=inf
  Enumerated Constant1 : simulink/Sources/Enumerated Constant  OutDataTypeStr=Enum: DoorsPositionTypes  Value=DoorsPositionTypes.DOORS_POS_ALL_DOORS_CLOSED  SampleTime=inf
  Enumerated Constant2 : simulink/Sources/Enumerated Constant  OutDataTypeStr=Enum: StateModeTypes  Value=StateModeTypes.STT_DISABLE  SampleTime=inf
  Enumerated Constant3 : simulink/Sources/Enumerated Constant  OutDataTypeStr=Enum: StateModeTypes  Value=StateModeTypes.STT_ENABLE  SampleTime=inf
  MATLAB Function : MATLAB Function  TreatAsAtomicUnit=on
  Multiport Switch : MultiPortSwitch  DataPortOrder=Zero-based contiguous  Inputs=2  zeroidx=on  SaturateOnIntegerOverflow=off  InputSameDT=off
  Relational Operator : RelationalOperator  Operator===  OutDataTypeStr=boolean  RndMeth=Simplest  InputSameDT=off
  Terminator : Terminator
  read_message_Cab_DC1 : TTlibrary/CAN/read_message_name  channel=IO_CAN_CHANNEL_1  id_format=IO_CAN_EXT_FRAME  get_msg_info=off  message_names=there is no CAN Unpack blocks  message_info=|  id=419319550  ac_mask=536870911  retranslation=off  io_error=on  sample_time=-1
      | Message Name: DC1
      |  Message ID Type: Extended (29-bit identifier)
      |  Message ID: 419319550
      settings: SourceProductName=TT control 500 series
  wires:
  CAN_Unpack_Cab_DC1/1 -> MATLAB Function/1(Value)
  read_message_Cab_DC1/1 -> CAN_Unpack_Cab_DC1/1  "msg_419319550"
  read_message_Cab_DC1/2 -> Terminator/1  "handler_err_419319550"
  Enumerated Constant2/1 -> Multiport Switch/2
  Multiport Switch/1 -> Data Store Write/1  "closedDoorSensState"
  Relational Operator/1 -> Multiport Switch/1
  Enumerated Constant/1 -> DataStoreWrite_PLC_StateM/1, Relational Operator/1
  Enumerated Constant1/1 -> Relational Operator/2
  Enumerated Constant3/1 -> Multiport Switch/3  "closedDoorSensState"

== system VCU_SW_1/InputLayer/InputNetwork/InputCCAN/GetCCAN100msec/Fan Rotation Direction Control  ==
  CAN_Unpack_Cab_FanRotationDirectionControl : canmsglib/CAN Unpack  MsgList=(none)  MsgName=FanRotationDirectionControl  MsgIDType=Extended (29-bit identifier)  MsgIdentifier=419375365  MsgLength=8  SignalInfo={ 'FanDirectCmd', '0', '2', 'LE', 'unsigned', 'Standard', '0', '1', '0', '0', '3'; 'FanReverseCmd', '2', '2', 'LE', 'unsigned', 'Standard', '0', '1', '0', '0', '3' }  IDPort=off  TimestampPort=off  ErrorPort=off  RemotePort=off  LengthPort=off  StatusPort=off  ApplyMinMax=off
  DataStoreWrite_PLC_StateM : DataStoreWrite  DataStoreName=InputNetworkData  DataStoreElements=InputNetworkData.CCAN.FanRotationDirectionControl.FanDirectCmd#InputNetworkData.CCAN.FanRotationDirectionControl.FanReverseCmd  IndexOptions=Index vector (dialog)  Indices=1  OutputSizes=1
  Function Caller1 : FunctionCaller  FunctionPrototype=rawValue = convUintPinToenumStt(uintValue)  InputArgumentSpecifications=<Enter example>  OutputArgumentSpecifications=<Enter example>
  Function Caller2 : FunctionCaller  FunctionPrototype=rawValue = convUintPinToenumStt(uintValue)  InputArgumentSpecifications=<Enter example>  OutputArgumentSpecifications=<Enter example>
  Terminator : Terminator
  read_message_Cab_FanRotationDirectionControl : TTlibrary/CAN/read_message_name  channel=IO_CAN_CHANNEL_1  id_format=IO_CAN_EXT_FRAME  get_msg_info=off  message_names=there is no CAN Unpack blocks  message_info=|  id=419375365  ac_mask=536870911  retranslation=off  io_error=on  sample_time=-1
      | Message Name: FanRotationDirectionControl
      |  Message ID Type: Extended (29-bit identifier)
      |  Message ID: 419375365
      settings: SourceProductName=TT control 500 series
  wires:
  Function Caller2/1 -> DataStoreWrite_PLC_StateM/2
  Function Caller1/1 -> DataStoreWrite_PLC_StateM/1
  CAN_Unpack_Cab_FanRotationDirectionControl/2 -> Function Caller2/1
  CAN_Unpack_Cab_FanRotationDirectionControl/1 -> Function Caller1/1
  read_message_Cab_FanRotationDirectionControl/1 -> CAN_Unpack_Cab_FanRotationDirectionControl/1  "msg_419375365"
  read_message_Cab_FanRotationDirectionControl/2 -> Terminator/1  "handler_err_419375365"

== system VCU_SW_1/InputLayer/InputNetwork/InputCCAN/GetCCAN100msec/Fan Rotation Direction Status  ==
  CAN_Unpack_Cab_FanRotationDirectionStatus : canmsglib/CAN Unpack  MsgList=(none)  MsgName=FanRotationDirectionStatus  MsgIDType=Extended (29-bit identifier)  MsgIdentifier=419377150  MsgLength=8  SignalInfo={ 'FanDirectSts', '0', '2', 'LE', 'unsigned', 'Standard', '0', '1', '0', '0', '3'; 'FanReverseSts', '2', '2', 'LE', 'unsigned', 'Standard', '0', '1', '0', '0', '3' }  IDPort=off  TimestampPort=off  ErrorPort=off  RemotePort=off  LengthPort=off  StatusPort=off  ApplyMinMax=off
  DataStoreWrite_PLC_StateM : DataStoreWrite  DataStoreName=InputNetworkData  DataStoreElements=InputNetworkData.CCAN.FanRotationDirectionStatus.FanDirectSts#InputNetworkData.CCAN.FanRotationDirectionStatus.FanReverseSts  IndexOptions=Index vector (dialog)  Indices=1  OutputSizes=1
  Function Caller1 : FunctionCaller  FunctionPrototype=rawValue = convUintPinToenumStt(uintValue)  InputArgumentSpecifications=<Enter example>  OutputArgumentSpecifications=<Enter example>
  Function Caller2 : FunctionCaller  FunctionPrototype=rawValue = convUintPinToenumStt(uintValue)  InputArgumentSpecifications=<Enter example>  OutputArgumentSpecifications=<Enter example>
  Terminator : Terminator
  read_message_Cab_FanRotationDirectionStatus : TTlibrary/CAN/read_message_name  channel=IO_CAN_CHANNEL_1  id_format=IO_CAN_EXT_FRAME  get_msg_info=off  message_names=there is no CAN Unpack blocks  message_info=|  id=419377150  ac_mask=536870911  retranslation=off  io_error=on  sample_time=-1
      | Message Name: FanRotationDirectionStatus
      |  Message ID Type: Extended (29-bit identifier)
      |  Message ID: 419377150
      settings: SourceProductName=TT control 500 series
  wires:
  Function Caller1/1 -> DataStoreWrite_PLC_StateM/2
  Function Caller2/1 -> DataStoreWrite_PLC_StateM/1
  CAN_Unpack_Cab_FanRotationDirectionStatus/2 -> Function Caller1/1
  CAN_Unpack_Cab_FanRotationDirectionStatus/1 -> Function Caller2/1
  read_message_Cab_FanRotationDirectionStatus/1 -> CAN_Unpack_Cab_FanRotationDirectionStatus/1  "msg_419377150"
  read_message_Cab_FanRotationDirectionStatus/2 -> Terminator/1  "handler_err_419377150"

== system VCU_SW_1/InputLayer/InputNetwork/InputCCAN/GetCCAN100msec/FuelTankAndFrameLock ==
  CAN_Unpack_Cab_FuelTankAndFrameLock : canmsglib/CAN Unpack  MsgList=(none)  MsgName=FuelTankAndFrameLock  MsgIDType=Extended (29-bit identifier)  MsgIdentifier=419375621  MsgLength=8  SignalInfo={ 'FrameLockCmd', '2', '2', 'LE', 'unsigned', 'Standard', '0', '1', '0', '-Inf', 'Inf'; 'FuelTankSwitch', '0', '2', 'LE', 'unsigned', 'Standard', '0', '1', '0', '0', '3' }  IDPort=off  TimestampPort=off  ErrorPort=off  RemotePort=off  LengthPort=off  StatusPort=off  ApplyMinMax=off
  Data Store Write : DataStoreWrite  DataStoreName=InputNetworkData  DataStoreElements=InputNetworkData.CCAN.FuelTankAndFrameLock.FrameLockCmd#InputNetworkData.CCAN.FuelTankAndFrameLock.FuelTankSwitch  IndexOptions=Index vector (dialog)  Indices=1  OutputSizes=1
  Terminator : Terminator
  read_message_Cab_FuelTankAndFrameLock : TTlibrary/CAN/read_message_name  channel=IO_CAN_CHANNEL_1  id_format=IO_CAN_EXT_FRAME  get_msg_info=off  message_names=there is no CAN Unpack blocks  message_info=|  id=419375621  ac_mask=536870911  retranslation=off  io_error=on  sample_time=-1
      | Message Name: OWWStatus
      |  Message ID Type: Extended (29-bit identifier)
      |  Message ID: 419376894
      settings: SourceProductName=TT control 500 series
  wires:
  read_message_Cab_FuelTankAndFrameLock/2 -> Terminator/1  "handler_err_419375621"
  read_message_Cab_FuelTankAndFrameLock/1 -> CAN_Unpack_Cab_FuelTankAndFrameLock/1  "msg_419375621"
  CAN_Unpack_Cab_FuelTankAndFrameLock/2 -> Data Store Write/2
  CAN_Unpack_Cab_FuelTankAndFrameLock/1 -> Data Store Write/1
